simulink model "DiagramaMalhaFechadaForno"  (R2015a)
settings: Solver=ode45  StartTime=0.0  StopTime=15000  RelTol=1e-3
undefined symbols (not defined in the file or in its folder): G
libraries: simulink x2
settings Model: Creator=Raian  LastModifiedBy=Emiliano

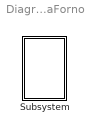
== system DiagramaMalhaFechadaForno ==
  Subsystem : Subsystem

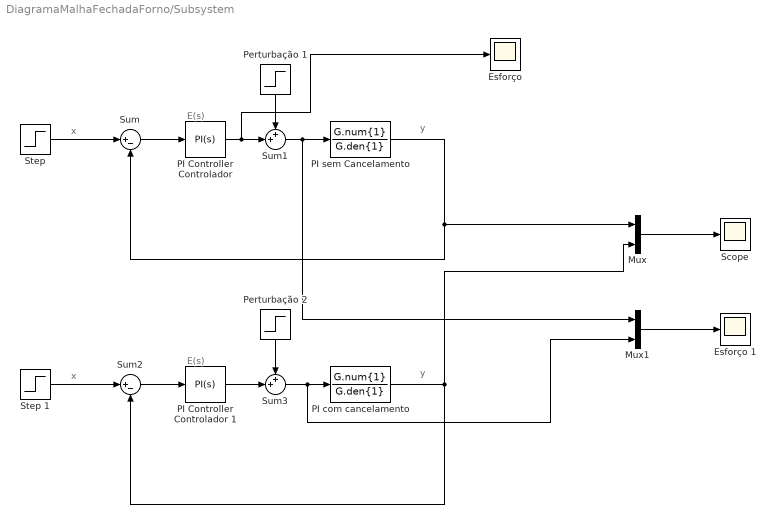
== system DiagramaMalhaFechadaForno/Subsystem ==
  note: E(s)
  note: x
  note: y
  note: E(s)
  note: x
  note: y
  "Esforço " : Scope
  Esforço 1 : Scope
      settings: ShowLegends=on  SaveName=ScopeData2
  Mux : Mux  Inputs=2
  Mux1 : Mux  Inputs=2
  "PI Controller Controlador " : simulink/Continuous/PID Controller  Controller=PI  TimeDomain=Continuous-time  SampleTime=-1  IntegratorMethod=Forward Euler  FilterMethod=Forward Euler  Form=Ideal  UseFilter=on  ControllerParametersSource=internal  P=0.01654  I=0.0001438  D=0  N=100  InitialConditionSource=internal  InitialConditionForIntegrator=0  InitialConditionForFilter=0  ExternalReset=none  LimitOutput=on  UpperSaturationLimit=1  LowerSaturationLimit=0  LinearizeAsGain=on  AntiWindupMode=clamping  Kb=1  TrackingMode=off  Kt=1  PParamMin=[]  PParamMax=[]  IParamMin=[]  IParamMax=[]  DParamMin=[]  DParamMax=[]  NParamMin=[]  NParamMax=[]  KbParamMin=[]  KbParamMax=[]  KtParamMin=[]  KtParamMax=[]  POutMin=[]  POutMax=[]  IOutMin=[]  IOutMax=[]  DOutMin=[]  DOutMax=[]  NOutMin=[]  NOutMax=[]  KbOutMin=[]  KbOutMax=[]  KtOutMin=[]  KtOutMax=[]  IntegratorOutMin=[]  IntegratorOutMax=[]  FilterOutMin=[]  FilterOutMax=[]  SumOutMin=[]  SumOutMax=[]  SumI1OutMin=[]  SumI1OutMax=[]  SumI2OutMin=[]  SumI2OutMax=[]  SumI3OutMin=[]  SumI3OutMax=[]  SumDOutMin=[]  SumDOutMax=[]  SaturationOutMin=[]  SaturationOutMax=[]  IntegratorContinuousStateAttributes=''  IntegratorStateMustResolveToSignalObject=off  IntegratorRTWStateStorageClass=Auto  FilterContinuousStateAttributes=''  FilterStateMustResolveToSignalObject=off  FilterRTWStateStorageClass=Auto  DifferentiatorICPrevScaledInput=0  DifferentiatorOutMin=[]  DifferentiatorOutMax=[]
  PI Controller Controlador 1 : simulink/Continuous/PID Controller  Controller=PI  TimeDomain=Continuous-time  SampleTime=-1  IntegratorMethod=Forward Euler  FilterMethod=Forward Euler  Form=Ideal  UseFilter=on  ControllerParametersSource=internal  P=0.0090  I=0.0001438  D=0  N=100  InitialConditionSource=internal  InitialConditionForIntegrator=0  InitialConditionForFilter=0  ExternalReset=none  LimitOutput=on  UpperSaturationLimit=1  LowerSaturationLimit=0  LinearizeAsGain=on  AntiWindupMode=clamping  Kb=1  TrackingMode=off  Kt=1  PParamMin=[]  PParamMax=[]  IParamMin=[]  IParamMax=[]  DParamMin=[]  DParamMax=[]  NParamMin=[]  NParamMax=[]  KbParamMin=[]  KbParamMax=[]  KtParamMin=[]  KtParamMax=[]  POutMin=[]  POutMax=[]  IOutMin=[]  IOutMax=[]  DOutMin=[]  DOutMax=[]  NOutMin=[]  NOutMax=[]  KbOutMin=[]  KbOutMax=[]  KtOutMin=[]  KtOutMax=[]  IntegratorOutMin=[]  IntegratorOutMax=[]  FilterOutMin=[]  FilterOutMax=[]  SumOutMin=[]  SumOutMax=[]  SumI1OutMin=[]  SumI1OutMax=[]  SumI2OutMin=[]  SumI2OutMax=[]  SumI3OutMin=[]  SumI3OutMax=[]  SumDOutMin=[]  SumDOutMax=[]  SaturationOutMin=[]  SaturationOutMax=[]  IntegratorContinuousStateAttributes=''  IntegratorStateMustResolveToSignalObject=off  IntegratorRTWStateStorageClass=Auto  FilterContinuousStateAttributes=''  FilterStateMustResolveToSignalObject=off  FilterRTWStateStorageClass=Auto  DifferentiatorICPrevScaledInput=0  DifferentiatorOutMin=[]  DifferentiatorOutMax=[]
  PI com cancelamento : TransferFcn  Numerator=G.num{1}  Denominator=G.den{1}
  "PI sem Cancelamento " : TransferFcn  Numerator=G.num{1}  Denominator=G.den{1}
  Perturbação 1 : Step  Time=5000  After=-0.1
  Perturbação 2 : Step  Time=5000  After=-0.1
  "Scope " : Scope
      settings: ShowLegends=on
  "Step " : Step  Time=0  After=250
  Step 1 : Step  Time=0  After=250
  Sum : Sum  Inputs=|+-
  Sum1 : Sum  Inputs=++|
  Sum2 : Sum  Inputs=|+-
  Sum3 : Sum  Inputs=++|
  wires:
  "Step "/1 -> Sum/1
  Sum/1 -> "PI Controller Controlador "/1
  "PI sem Cancelamento "/1 -> Mux/1, Sum/2
  Sum1/1 -> "PI sem Cancelamento "/1, Mux1/1
  Perturbação 1/1 -> Sum1/1
  "PI Controller Controlador "/1 -> "Esforço "/1, Sum1/2
  Step 1/1 -> Sum2/1
  Sum2/1 -> PI Controller Controlador 1/1
  PI com cancelamento/1 -> Mux/2, Sum2/2
  Sum3/1 -> Mux1/2, PI com cancelamento/1
  Perturbação 2/1 -> Sum3/1
  PI Controller Controlador 1/1 -> Sum3/2
  Mux/1 -> "Scope "/1
  Mux1/1 -> Esforço 1/1
